simulink model "Correccion_Sist_Fisico"  (R2021a)
settings: Solver=VariableStepAuto  StartTime=0.0  StopTime=inf  RelTol=1e-3
values from neighbouring files (symbols this model uses):
  b_cx = 1*10^6    (= 1000000)    [parametros.m]
  b_cy = 1*10^7    (= 10000000)    [parametros.m]
  b_eq = (b_td+b_tm*(r_t^2))/r_td    (= 10803.6)    [parametros.m]
  b_eqh = 2*(b_hd+b_hm*(r_h^2))/r_hd    (= 23253.3333333)    [parametros.m]
  b_ha = b_eqh/r_h - n_h*w_posh*(J_eqh + 0.5*m_l_*r_hd)/r_h    [parametros.m]
  b_hb = 1*10^8    (= 100000000)    [parametros.m]
  b_hEb = 2.2*10^9    (= 2200000000)    [parametros.m]
  b_t = 90    [parametros.m]
  b_ta = n_t*w_post*(r_td*J_eqt/r_t) - r_td*b_eqt/r_t    [parametros.m]
  b_tb = 5*10^6    (= 5000000)    [parametros.m]
  b_tw = 3*10^3    (= 3000)    [parametros.m]
  b_wu = 150    [parametros.m]
  g = 9.80665    [parametros.m]
  H_c = 2.5    [parametros.m]
  J_eq = (J_td+J_tm_tb*(r_t^2))/r_td    (= 15000)    [parametros.m]
  J_eqh = 2*(J_hd_hEb+J_hm_hb*(r_h^2))/r_hd    (= 48853.3333333)    [parametros.m]
  K_cy = 1.8*10^9    (= 1800000000)    [parametros.m]
  K_hsa = -n_h*(w_posh^2)*(J_eqh + 0.5*m_l_*r_hd)/r_t    [parametros.m]
  K_hsia = -(w_posh^3)*(J_eqh + 0.5*m_l_*r_hd)/r_t    [parametros.m]
  K_tsa = n_t*(w_post^2)*J_eqt*r_td/r_t    [parametros.m]
  K_tsia = (w_post^3)*J_eqt*r_td/r_t    [parametros.m]
  K_tw = 4.8*10^5    (= 480000)    [parametros.m]
  k_wu = 2.36*10^8    (= 236000000)    [parametros.m]
  lh_inicial = 45-yl_inicial    (= 40)    [parametros.m]
  M_c_MAX = 50000 + M_s    (= 65000)    [parametros.m]
  M_real = 10000    [parametros.m]
  M_s = 15000    [parametros.m]
  M_t = 30000    [parametros.m]
  r_h = 22    [parametros.m]
  r_hd = 0.75    [parametros.m]
  r_t = 30    [parametros.m]
  r_td = 0.5    [parametros.m]
  T_hb_MAX = 5*10^4    (= 50000)    [parametros.m]
  T_hEb_MAX = 1.1*10^6    (= 1100000)    [parametros.m]
  T_hm_MAX = 2*10^4    (= 20000)    [parametros.m]
  T_s2 = 5e-3    (= 0.005)    [parametros.m]
  T_tb_MAX = 5*10^3    (= 5000)    [parametros.m]
  T_tm_MAX = 3*10^3    (= 3000)    [parametros.m]
  tau_hm = 1.0e-2    (= 0.01)    [parametros.m]
  tau_tm = 1.0e-2    (= 0.01)    [parametros.m]
  TensionMinima = (M_s*g/2)*0.5    (= 36774.9375)    [parametros.m]
  v_h_MAX_c = +1.5    (= 1.5)    [parametros.m]
  v_t_MAX = +4    (= 4)    [parametros.m]
  v_t_MIN = -4    [parametros.m]
  w_hm_min = pi/4    (= 0.785398163397)    [parametros.m]
  w_tm_min = pi/4    (= 0.785398163397)    [parametros.m]
  xt_inicial = -10    [parametros.m]
  Y_t0 = 45    [parametros.m]
  yl_inicial = 5    [parametros.m]
undefined symbols (not defined in the file or in its folder): DiscIntNeverNeededParam
libraries: simulink x10, dspstat3 x1, vrlib x1
(part 1 of 3)
settings Model: Creator=aguss  LastModifiedBy=aguss
settings SolverCC: ZeroCrossAlgorithm=Adaptive
settings DebuggingCC: IgnoredZcDiagnostic=none

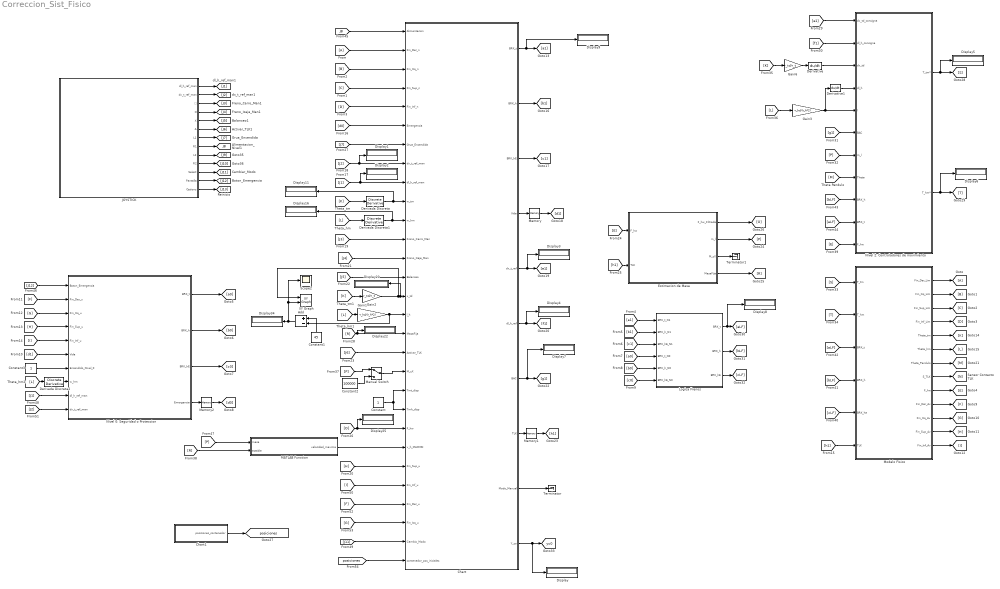
== system Correccion_Sist_Fisico ==
  Add : Sum  Inputs=+-
  Chart : Stateflow chart  TreatAsAtomicUnit=on
      settings: PortSchema="{\"entries\":[{\"content\":{\"sides\":[{\"content\":{\"connectorIds\":[\"In1\",\"In2\",\"In3\",\"In4\",\"In5\",\"In6\",\"In7\",\"In8\",\"In9\",\"In10\",\"In11\",\"In12\",\"In13\",\"In14\",\"In15\",\"In16\",\"In17\",\"In18\",\"In19\",\"In20\",\"In21\",\"In22\",\"In23\",\"In24\",\"In25\",\"In28\",\"In27\",\"In26\",\"In29\"]},\"type\":\"ConnectorPlacement.EquallySpacedRectSide\",\"uuid\":\"54a235bb-383c-4b33-a4d9-6e61ae54fc2f\"},{\"content\":{\"connectorIds\":[\"Out1\",\"Out2\",\"Out3\",\"Out4\",\"Out5\",\"Out6\",\"Out7\",\"Out8\",\"Out9\",\"Out10\"],\"side\":\"RIGHT\"},\"type\":\"ConnectorPlacement.EquallySpacedRectSide\",\"uuid\":\"22d5bc5e-44c7-4d0f-b301-3d6b5a5c05fa\"},{\"content\":{\"connectorIds\":[],\"side\":\"TOP\"},\"type\":\"ConnectorPlacement.EquallySpacedRectSide\",\"uuid\":\"f8e7191e-c2be-47a5-9ee2-638adab41de6\"},{\"content\":{\"connectorIds\":[],\"side\":\"BOTTOM\"},\"type\":\"ConnectorPlacement.EquallySpacedRectSide\",\"uuid\":\"c3fe6b96-a7cd-4655-bccb-6e03a1555df7\"}]},\"type\":\"ConnectorPlacement.EquallySpacedConnector\",\"uuid\":\"917daf47-55d7-4e55-b1eb-670cdd820ed3\"}],\"packageUris\":[\"http://schema.mathworks.com/mf0/Connector/R2020b\"],\"version\":\"1.0\"}"
  Chart1 : Stateflow chart  TreatAsAtomicUnit=on
  Constant : Constant
  Constant1 : Constant  Value=45
  Constant2 : Constant  Value=100000
  Constant3 : Constant
  Derivada Discreta : simulink/Discrete/Discrete Derivative  gainval=1.0  ICPrevScaledInput=0.0  OutMin=[]  OutMax=[]  OutDataType=fixdt(1, 16)  OutScaling=2^-10  DoSatur=off
  Derivada Discreta1 : simulink/Discrete/Discrete Derivative  gainval=1.0  ICPrevScaledInput=0.0  OutMin=[]  OutMax=[]  OutDataType=fixdt(1, 16)  OutScaling=2^-10  DoSatur=off
  Derivada Discreta2 : simulink/Discrete/Discrete Derivative  gainval=1.0  ICPrevScaledInput=0.0  OutMin=[]  OutMax=[]  OutDataType=fixdt(1, 16)  OutScaling=2^-10  DoSatur=off
  Derivative : Derivative
  Derivative1 : Derivative
  Display{,1..9,11,16,20,22,25,34} (16 alike) : Display
  Estimacion de Masa : Subsystem
  Gain1 : Gain  Gain=-r_hd/(r_h*2)
  Gain2 : Gain  Gain=r_td/r_t
  Gain3 : Gain  Gain=-r_hd/(r_h*2)
  Gain6 : Gain  Gain=r_td/r_t
  JOYSTICK : Subsystem
  Logica Frenos : Subsystem
  MATLAB Function : MATLAB Function  TreatAsAtomicUnit=on
  Manual Switch : ManualSwitch
  Memory : Memory
  Memory1 : Memory
  Memory2 : Memory
  Modelo Físico : Subsystem
  Nivel 0: Seguridad o Proteccion : Stateflow chart  TreatAsAtomicUnit=on
  Nivel 2: Controladores de movimiento : Subsystem
  Scope2 : Scope
  Terminator : Terminator
  Terminator1 : Terminator
  XY Graph : simulink/Sinks/XY Graph  xmin=-32  xmax=52  ymin=-22  ymax=42  st=-1
  tag scope: J8=global, posiciones=global, yc0=global
  wires:
  Modelo Físico/5(Theta_tm) -> [K]
  Modelo Físico/6(Theta_hm) -> [L]
  Modelo Físico/10(Fin_Der_Av) -> [F]
  Modelo Físico/7(Theta_Pendulo) -> [M]
  Modelo Físico/2(Fin_Izq_Lim) -> [B]
  Modelo Físico/8(S_TLK) -> [N]
  Modelo Físico/3(Fin_Sup_Lim) -> [C]
  Modelo Físico/1(Fin_Der_Lim) -> [A]
  Modelo Físico/9(F_hw) -> [E]
  Modelo Físico/4(Fin_Inf_Lim) -> [D]
  Modelo Físico/11(Fin_Izq_Av) -> [G]
  Modelo Físico/12(Fin_Sup_Av) -> [H]
  Modelo Físico/13(Fin_Inf_Av) -> [I]
  [B] -> Chart/3(Fin_Izq_n)
  [A] -> Chart/2(Fin_Der_n)
  Constant/1 -> Chart/20(Tmt_disp), Chart/21(Tmh_disp)
  [J8] -> Chart/1(Alimentacion)
  [C] -> Chart/4(Fin_Sup_n)
  [D] -> Chart/5(Fin_Inf_n)
  [J7] -> Chart/7(Grua_Encendida)
  Derivada Discreta1/1 -> Display16/1, Chart/11(w_hm)
  Derivada Discreta/1 -> Chart/10(w_tm), Display11/1
  Gain2/1 -> Display20/1, Chart/15(x_td), XY Graph/1
  MATLAB Function/1(velocidad_maxima) -> Chart/23(v_h_MAXMIN)
  JOYSTICK/13(Options) -> [J13]
  JOYSTICK/9(L2) -> [J9]
  JOYSTICK/12(Pantalla) -> [J12]
  JOYSTICK/4(O) -> [J4]
  JOYSTICK/1(dl_h_ref_man) -> [J1]
  JOYSTICK/6(Δ) -> [J6]
  JOYSTICK/5(X) -> [J5]
  JOYSTICK/10(R2) -> [J10]
  JOYSTICK/2(dx_t_ref_man) -> [J2]
  JOYSTICK/11(Select) -> [J11]
  JOYSTICK/8(R1) -> [J8]
  JOYSTICK/3(☐) -> [J3]
  JOYSTICK/7(L1) -> [J7]
  Chart/9(Modo_Manual) -> Terminator/1
  Nivel 0: Seguridad o Proteccion/1(BRK_t) -> [a0]
  Nivel 0: Seguridad o Proteccion/2(BRK_h) -> [b0]
  Nivel 0: Seguridad o Proteccion/3(BRK_hE) -> [c0]
  Nivel 0: Seguridad o Proteccion/4(Emergencia) -> Memory2/1
  [a1] -> Logica Frenos/1(BRK_t_N1)
  [b1] -> Logica Frenos/2(BRK_h_N1)
  [c1] -> Logica Frenos/3(BRK_hE_N1)
  [a0] -> Logica Frenos/4(BRK_t_N0)
  [b0] -> Logica Frenos/5(BRK_h_N0)
  [c0] -> Logica Frenos/6(BRK_hE_N0)
  Chart/4(Vida) -> Memory/1
  [d1] -> Nivel 0: Seguridad o Proteccion/6(Vida)
  [F] -> Nivel 0: Seguridad o Proteccion/2(Fin_Der_u)
  [G] -> Nivel 0: Seguridad o Proteccion/3(Fin_Izq_u)
  [I] -> Nivel 0: Seguridad o Proteccion/5(Fin_Inf_u)
  Constant3/1 -> Nivel 0: Seguridad o Proteccion/7(Encendido_Nivel_0)
  Chart/8(TLK) -> Memory1/1
  [h1] -> Modelo Físico/6(TLK)
  [E] -> Estimacion de Masa/1(F_hw)
  [h1] -> Estimacion de Masa/2(TLK)
  Estimacion de Masa/2(m_l) -> [P]
  [f1] -> Nivel 2: Controladores de movimiento/2(dl_h_consigna)
  [e1] -> Nivel 2: Controladores de movimiento/1(dx_td_consigna)
  [g1] -> Nivel 2: Controladores de movimiento/6(BAC)
  [P] -> Nivel 2: Controladores de movimiento/7(m_l)
  Nivel 2: Controladores de movimiento/2(T_hm*) -> Display6/1, [T]
  Nivel 2: Controladores de movimiento/1(T_tm*) -> Display5/1, [S]
  [S] -> Modelo Físico/1(T_tm)
  [T] -> Modelo Físico/2(T_hm)
  [K] -> Gain6/1
  Gain6/1 -> Derivative/1
  [L] -> Gain3/1
  Gain3/1 -> Derivative1/1, Nivel 2: Controladores de movimiento/5(l)
  Derivative1/1 -> Nivel 2: Controladores de movimiento/4(dl_h)
  [M] -> Nivel 2: Controladores de movimiento/8(Theta)
  Memory/1 -> [d1]
  Memory1/1 -> [h1]
  Memory2/1 -> [d0]
  Estimacion de Masa/4(MasaFija) -> [R]
  Chart/6(dl_h_ref) -> Display4/1, [f1]
  Chart/5(dx_t_ref) -> Display3/1, [e1]
  [P] -> MATLAB Function/1(masa)
  [K] -> Derivada Discreta/1
  [d0] -> Chart/6(Emergencia)
  [J1] -> Display2/1, Chart/9(dl_h_ref_man)
  [J2] -> Display1/1, Chart/8(dx_t_ref_man)
  [J5] -> Chart/14(Balanceo)
  [L] -> Derivada Discreta1/1
  [J4] -> Chart/13(Freno_Izaje_Man)
  [J3] -> Chart/12(Freno_Carro_Man)
  [J6] -> Chart/18(Activar_TLK)
  [K] -> Gain2/1
  [R] -> Chart/17(MasaFija), Display22/1
  [L] -> Gain1/1
  [O] -> Chart/22(F_hw), Display25/1
  Chart/7(BAC) -> Display7/1, [g1]
  Chart/3(BRK_hE) -> [c1]
  Chart/2(BRK_h) -> [b1]
  [P] -> Manual Switch/1
  [R] -> MATLAB Function/2(estable)
  [E] -> Nivel 2: Controladores de movimiento/11(F_hw)
  Logica Frenos/1(BRK_t) -> Display8/1, [aLF]
  Logica Frenos/2(BRK_h) -> [bLF]
  Logica Frenos/3(BRK_hE) -> [cLF]
  [aLF] -> Modelo Físico/3(BRK_t)
  [bLF] -> Modelo Físico/4(BRK_h)
  [cLF] -> Modelo Físico/5(BRK_he)
  [aLF] -> Nivel 2: Controladores de movimiento/10(BRK_t)
  [bLF] -> Nivel 2: Controladores de movimiento/9(BRK_h)
  [J12] -> Nivel 0: Seguridad o Proteccion/1(Boton_Emergencia)
  [L] -> Derivada Discreta2/1
  Derivada Discreta2/1 -> Nivel 0: Seguridad o Proteccion/8(w_hm)
  Gain1/1 -> Chart/16(l_h), Add/2
  Add/1 -> XY Graph/2, Scope2/1, Display34/1
  Constant1/1 -> Add/1
  [H] -> Nivel 0: Seguridad o Proteccion/4(Fin_Sup_u)
  [H] -> Chart/24(Fin_Sup_u)
  [J1] -> Nivel 0: Seguridad o Proteccion/9(dl_h_ref_man)
  [J11] -> Chart/26(Cambio_Modo)
  [I] -> Chart/25(Fin_Inf_u)
  [J2] -> Nivel 0: Seguridad o Proteccion/10(dx_t_ref_man)
  [F] -> Chart/28(Fin_Der_u)
  [G] -> Chart/27(Fin_Izq_u)
  Derivative/1 -> Nivel 2: Controladores de movimiento/3(dx_td)
  Manual Switch/1 -> Chart/19(M_cX)
  Constant2/1 -> Manual Switch/2
  Estimacion de Masa/1(F_hw_Filtrada) -> [O]
  Estimacion de Masa/3(M_cX) -> Terminator1/1
  Chart1/1(posiciones_contenedor) -> [posiciones]
  [posiciones] -> Chart/29(contenedor_pos_iniciales)
  Chart/10(Y_co) -> Display/1, [yc0]
  Chart/1(BRK_t) -> Display9/1, [a1]

== system Correccion_Sist_Fisico/Estimacion de Masa ==
  F_hw : Inport
  TLK : Inport  Port=2
  Discrete Derivative1 : simulink/Discrete/Discrete Derivative  gainval=1.0  ICPrevScaledInput=0.0  OutMin=[]  OutMax=[]  OutDataType=fixdt(1, 16)  OutScaling=2^-10  DoSatur=off
  Leaky integrator : Subsystem
  MATLAB Function1 : MATLAB Function  TreatAsAtomicUnit=on
  Moving Average2 : dspstat3/Moving Average  Method=Sliding window  ForgettingFactorPort=off  SpecifyWindowLength=on  WindowLength=4  ForgettingFactor=0.9  SimulateUsing=Code generation
  Zero-Order Hold : ZeroOrderHold  SampleTime=-1
  F_hw_Filtrada : Outport
  m_l : Outport  Port=2
  M_cX : Outport  Port=3
  MasaFija : Outport  Port=4
  wires:
  Moving Average2/1 -> Discrete Derivative1/1, Zero-Order Hold/1
  Discrete Derivative1/1 -> MATLAB Function1/2(dF_hw)
  TLK/1 -> MATLAB Function1/3(TLK)
  F_hw/1 -> Leaky integrator/1(Entrada)
  MATLAB Function1/1(m_l) -> m_l/1
  MATLAB Function1/2(M_cX) -> M_cX/1
  MATLAB Function1/3(MasaFija) -> MasaFija/1
  Leaky integrator/1(Salida) -> Moving Average2/1
  Zero-Order Hold/1 -> F_hw_Filtrada/1, MATLAB Function1/1(tension)

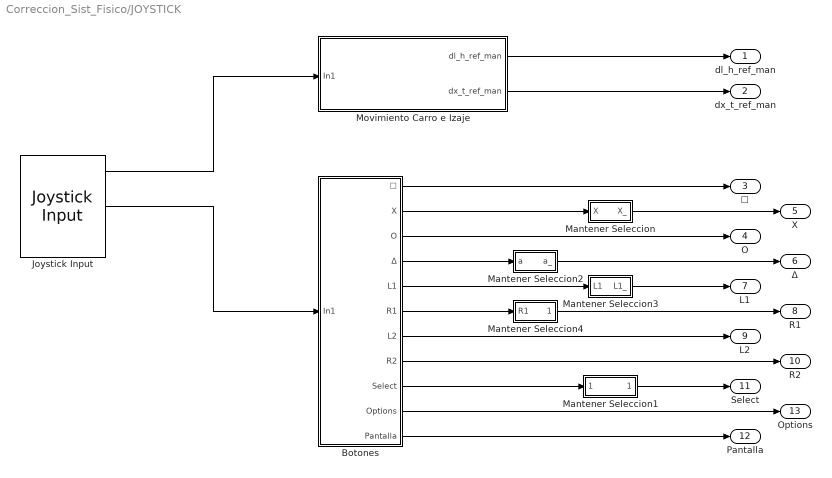
== system Correccion_Sist_Fisico/JOYSTICK ==
  Botones : Subsystem
  Joystick Input : vrlib/Joystick Input  joyid=1  adjustports=on  forcefeed=off
  Mantener Seleccion : Stateflow chart  TreatAsAtomicUnit=on
  Mantener Seleccion1 : Stateflow chart  TreatAsAtomicUnit=on
  Mantener Seleccion2 : Stateflow chart  TreatAsAtomicUnit=on
  Mantener Seleccion3 : Stateflow chart  TreatAsAtomicUnit=on
  Mantener Seleccion4 : Stateflow chart  TreatAsAtomicUnit=on
  Movimiento Carro e Izaje : Subsystem
  dl_h_ref_man : Outport
  dx_t_ref_man : Outport  Port=2
  ☐ : Outport  Port=3
  O : Outport  Port=4
  X : Outport  Port=5
  Δ : Outport  Port=6
  L1 : Outport  Port=7
  R1 : Outport  Port=8
  L2 : Outport  Port=9
  R2 : Outport  Port=10
  Select : Outport  Port=11
  Pantalla : Outport  Port=12
  Options : Outport  Port=13
  wires:
  Joystick Input/1 -> Movimiento Carro e Izaje/1(In1)
  Movimiento Carro e Izaje/1(dl_h_ref_man) -> dl_h_ref_man/1
  Movimiento Carro e Izaje/2(dx_t_ref_man) -> dx_t_ref_man/1
  Joystick Input/2 -> Botones/1(In1)
  Botones/1(☐) -> ☐/1
  Botones/2(X) -> Mantener Seleccion/1(X)
  Botones/3(O) -> O/1
  Botones/4(Δ) -> Mantener Seleccion2/1(a)
  Botones/5(L1) -> Mantener Seleccion3/1(L1)
  Botones/6(R1) -> Mantener Seleccion4/1(R1)
  Botones/7(L2) -> L2/1
  Botones/8(R2) -> R2/1
  Botones/9(Select) -> Mantener Seleccion1/1(Select)
  Botones/10(Options) -> Options/1
  Botones/11(Pantalla) -> Pantalla/1
  Mantener Seleccion/1(X_) -> X/1
  Mantener Seleccion2/1(a_) -> Δ/1
  Mantener Seleccion3/1(L1_) -> L1/1
  Mantener Seleccion4/1(R1_) -> R1/1
  Mantener Seleccion1/1(Select_) -> Select/1

== system Correccion_Sist_Fisico/Logica Frenos ==
  BRK_t_N1 : Inport
  BRK_h_N1 : Inport  Port=2
  BRK_hE_N1 : Inport  Port=3
  BRK_t_N0 : Inport  Port=4
  BRK_h_N0 : Inport  Port=5
  BRK_hE_N0 : Inport  Port=6
  AND : Logic  IconShape=distinctive  AllPortsSameDT=off  OutDataTypeStr=boolean
  AND1 : Logic  IconShape=distinctive  AllPortsSameDT=off  OutDataTypeStr=boolean
  AND2 : Logic  IconShape=distinctive  AllPortsSameDT=off  OutDataTypeStr=boolean
  BRK_t : Outport
  BRK_h : Outport  Port=2
  BRK_hE : Outport  Port=3
  wires:
  AND/1 -> BRK_h/1
  BRK_h_N1/1 -> AND/1
  BRK_h_N0/1 -> AND/2
  AND1/1 -> BRK_t/1
  BRK_t_N1/1 -> AND1/1
  BRK_t_N0/1 -> AND1/2
  AND2/1 -> BRK_hE/1
  BRK_hE_N1/1 -> AND2/1
  BRK_hE_N0/1 -> AND2/2

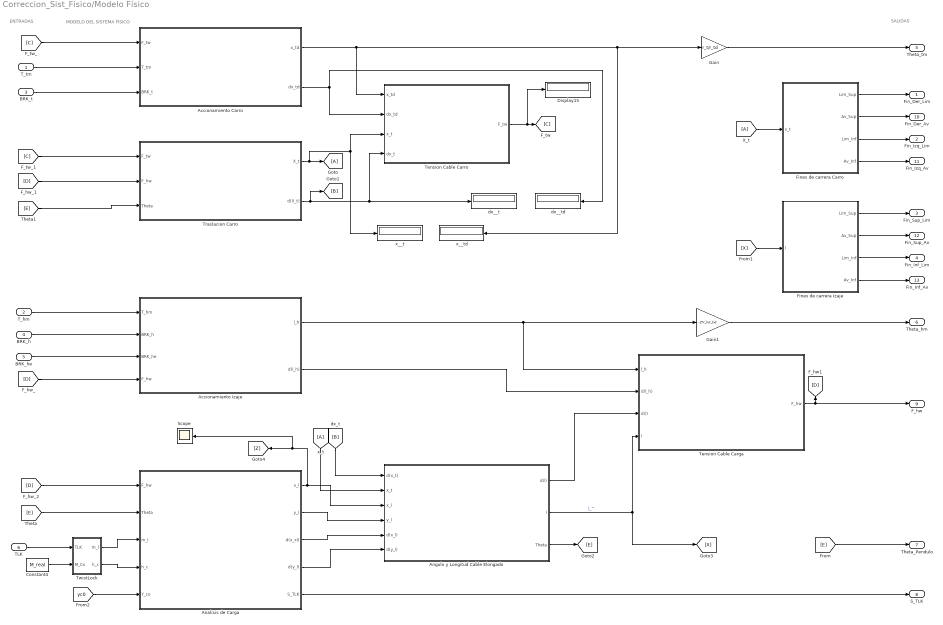
== system Correccion_Sist_Fisico/Modelo Físico ==
  note: SALIDAS
  note: MODELO DEL SISTEMA FÍSICO
  note: ENTRADAS
  T_tm : Inport
  T_hm : Inport  Port=2
  BRK_t : Inport  Port=3
  BRK_h : Inport  Port=4
  BRK_he : Inport  Port=5
  TLK : Inport  Port=6
  Accionamiento Carro : Subsystem
  Accionamiento Izaje : Subsystem
  Analisis de Carga : Subsystem
  Angulo y Longitud Cable Elongado : Subsystem
  Constant4 : Constant  Value=M_real
  Display15 : Display
  Fines de carrera Carro : Subsystem
  Fines de carrera Izaje : Subsystem
  Gain : Gain  Gain=r_t/r_td
  Gain1 : Gain  Gain=-2*r_h/r_hd
  Scope : Scope
  Tension Cable Carga : Subsystem
  Tension Cable Carro : Subsystem
  Traslacion Carro : Subsystem
  TwistLock : Subsystem
  dx__t : Display
  dx__td : Display
  x__t : Display
  x__td : Display
  Fin_Der_Lim : Outport
  Fin_Izq_Lim : Outport  Port=2
  Fin_Sup_Lim : Outport  Port=3
  Fin_Inf_Lim : Outport  Port=4
  Theta_tm : Outport  Port=5
  Theta_hm : Outport  Port=6
  Theta_Pendulo : Outport  Port=7
  S_TLK : Outport  Port=8
  F_hw : Outport  Port=9
  Fin_Der_Av : Outport  Port=10
  Fin_Izq_Av : Outport  Port=11
  Fin_Sup_Av : Outport  Port=12
  Fin_Inf_Av : Outport  Port=13
  wires:
  Analisis de Carga/5(S_TLK) -> S_TLK/1
  Fines de carrera Carro/3(Lim_Inf) -> Fin_Izq_Lim/1
  Traslacion Carro/1(X_t) -> Tension Cable Carro/3(x_t), x__t/1, [A]
  Fines de carrera Izaje/2(Av_Sup) -> Fin_Sup_Av/1
  [D] -> Accionamiento Izaje/4(F_hw)
  Angulo y Longitud Cable Elongado/3(Theta) -> [E]
  T_tm/1 -> Accionamiento Carro/2(T_tm)
  Tension Cable Carga/1(F_hw) -> F_hw/1, [D]
  TwistLock/1(m_l) -> Analisis de Carga/3(m_l)
  [E] -> Analisis de Carga/2(Theta)
  Accionamiento Izaje/1(l_h) -> Gain1/1, Tension Cable Carga/1(l_h)
  BRK_t/1 -> Accionamiento Carro/3(BRK_t)
  Fines de carrera Carro/1(Lim_Sup) -> Fin_Der_Lim/1
  Accionamiento Carro/1(x_td) -> x__td/1, Gain/1, Tension Cable Carro/1(x_td)
  Fines de carrera Izaje/3(Lim_Inf) -> Fin_Inf_Lim/1
  Analisis de Carga/2(y_l) -> Angulo y Longitud Cable Elongado/4(y_l)
  TwistLock/2(h_c) -> Analisis de Carga/4(h_c)
  BRK_h/1 -> Accionamiento Izaje/2(BRK_h)
  Fines de carrera Carro/2(Av_Sup) -> Fin_Der_Av/1
  [D] -> Analisis de Carga/1(F_hw)
  Accionamiento Carro/2(dx_td) -> Tension Cable Carro/2(dx_td), dx__td/1
  Tension Cable Carro/1(F_tw) -> Display15/1, [C]
  T_hm/1 -> Accionamiento Izaje/1(T_hm)
  [C] -> Accionamiento Carro/1(F_tw)
  [E] -> Theta_Pendulo/1
  Traslacion Carro/2(d(X_t)) -> Tension Cable Carro/4(dx_t), dx__t/1, [B]
  [D] -> Traslacion Carro/2(F_hw)
  Fines de carrera Izaje/4(Av_Inf) -> Fin_Inf_Av/1
  Angulo y Longitud Cable Elongado/1(d(l)) -> Tension Cable Carga/3(d(l))
  TLK/1 -> TwistLock/1(TLK)
  [E] -> Traslacion Carro/3(Theta)
  Accionamiento Izaje/2(d(l_h)) -> Tension Cable Carga/2(d(l_h))
  Fines de carrera Izaje/1(Lim_Sup) -> Fin_Sup_Lim/1
  Gain1/1 -> Theta_hm/1
  Fines de carrera Carro/4(Av_Inf) -> Fin_Izq_Av/1
  [B] -> Angulo y Longitud Cable Elongado/1(d(x_t))
  Analisis de Carga/3(d(x_xl)) -> Angulo y Longitud Cable Elongado/5(d(x_l))
  Analisis de Carga/4(d(y_l)) -> Angulo y Longitud Cable Elongado/6(d(y_l))
  Gain/1 -> Theta_tm/1
  [C] -> Traslacion Carro/1(F_tw)
  [A] -> Angulo y Longitud Cable Elongado/2(x_t)
  [A] -> Fines de carrera Carro/1(x_t)
  BRK_he/1 -> Accionamiento Izaje/3(BRK_he)
  [X] -> Fines de carrera Izaje/1(l)
  Analisis de Carga/1(x_l) -> Angulo y Longitud Cable Elongado/3(x_l), Scope/1, [Z]
  Angulo y Longitud Cable Elongado/2(l) -> Tension Cable Carga/4(l), [X]  "l_^"
  Constant4/1 -> TwistLock/2(M_Cx)
  [yc0] -> Analisis de Carga/5(Y_co)

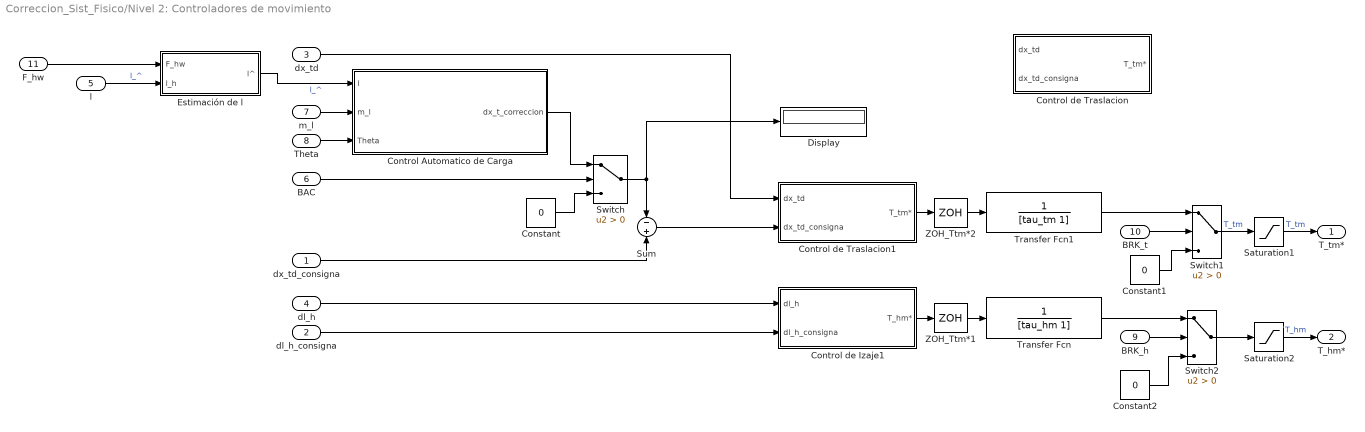
== system Correccion_Sist_Fisico/Nivel 2: Controladores de movimiento ==
  dx_td_consigna : Inport
  dl_h_consigna : Inport  Port=2
  dx_td : Inport  Port=3
  dl_h : Inport  Port=4
  l : Inport  Port=5
  BAC : Inport  Port=6
  m_l : Inport  Port=7
  Theta : Inport  Port=8
  BRK_h : Inport  Port=9
  BRK_t : Inport  Port=10
  F_hw : Inport  Port=11
  Constant : Constant  Value=0
  Constant1 : Constant  Value=0
  Constant2 : Constant  Value=0
  Control Automatico de Carga : Subsystem
  Control de Izaje1 : Subsystem
  Control de Traslacion : Subsystem
  Control de Traslacion1 : Subsystem
  Display : Display
  Estimación de l : Subsystem
  Saturation1 : Saturate  UpperLimit=T_tm_MAX  LowerLimit=-T_tm_MAX
  Saturation2 : Saturate  UpperLimit=T_hm_MAX  LowerLimit=-T_hm_MAX
  Sum : Sum  Inputs=-+
  Switch : Switch  Criteria=u2 > Threshold
  Switch1 : Switch  Criteria=u2 > Threshold
  Switch2 : Switch  Criteria=u2 > Threshold
  Transfer Fcn : TransferFcn  Denominator=[tau_hm 1]
  Transfer Fcn1 : TransferFcn  Denominator=[tau_tm 1]
  ZOH_Ttm*1 : ZeroOrderHold  SampleTime=T_s2
  ZOH_Ttm*2 : ZeroOrderHold  SampleTime=T_s2
  T_tm* : Outport
  T_hm* : Outport  Port=2
  wires:
  Control de Izaje1/1(T_hm*) -> ZOH_Ttm*1/1
  dx_td_consigna/1 -> Sum/2
  dx_td/1 -> Control de Traslacion1/1(dx_td)
  dl_h/1 -> Control de Izaje1/1(dl_h)
  dl_h_consigna/1 -> Control de Izaje1/2(dl_h_consigna)
  Sum/1 -> Control de Traslacion1/2(dx_td_consigna)
  Control Automatico de Carga/1(dx_t_correccion) -> Switch/1
  Constant/1 -> Switch/3
  Switch/1 -> Sum/1, Display/1
  BAC/1 -> Switch/2
  Theta/1 -> Control Automatico de Carga/3(Theta)
  m_l/1 -> Control Automatico de Carga/2(m_l)
  Transfer Fcn1/1 -> Switch1/1
  Switch2/1 -> Saturation2/1
  Switch1/1 -> Saturation1/1  "T_tm"
  Transfer Fcn/1 -> Switch2/1
  BRK_h/1 -> Switch2/2
  BRK_t/1 -> Switch1/2
  Saturation2/1 -> T_hm*/1  "T_hm"
  F_hw/1 -> Estimación de l/1(F_hw)
  l/1 -> Estimación de l/2(l_h)  "l_^"
  Estimación de l/1(l^) -> Control Automatico de Carga/1(l)  "l_^"
  Constant1/1 -> Switch1/3
  Constant2/1 -> Switch2/3
  Control de Traslacion1/1(T_tm*) -> ZOH_Ttm*2/1
  ZOH_Ttm*1/1 -> Transfer Fcn/1
  ZOH_Ttm*2/1 -> Transfer Fcn1/1
  Saturation1/1 -> T_tm*/1  "T_tm"

== system Correccion_Sist_Fisico/Estimacion de Masa/Leaky integrator ==
  Entrada : Inport
  Constant17 : Constant
  Delay1 : Delay  DelayLength=1  InitialCondition=0
  Divide1 : Product  Inputs=*/
  M : Constant  Value=100
  Product2 : Product
  Product3 : Product
  Sum1 : Sum  Inputs=|+-
  Sum2 : Sum  Inputs=|-+
  Sum5 : Sum  Inputs=|++
  Salida : Outport
  wires:
  Sum5/1 -> Salida/1, Delay1/1
  M/1 -> Sum2/2, Divide1/2
  Constant17/1 -> Sum2/1, Sum1/1
  Sum1/1 -> Product2/2
  Product2/1 -> Sum5/1
  Delay1/1 -> Product3/1
  Divide1/1 -> Product3/2, Sum1/2
  Product3/1 -> Sum5/2
  Sum2/1 -> Divide1/1
  Entrada/1 -> Product2/1

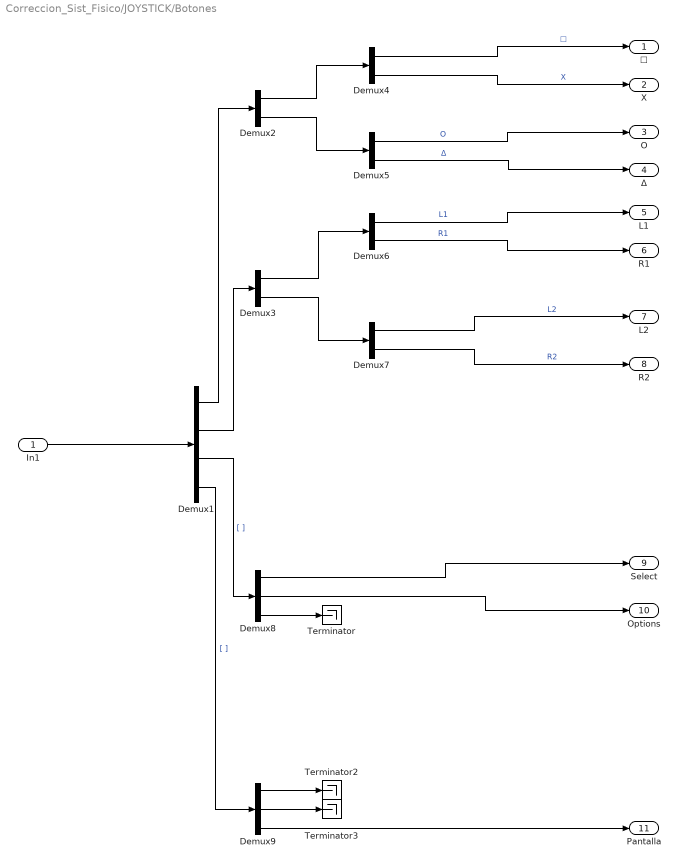
== system Correccion_Sist_Fisico/JOYSTICK/Botones ==
  In1 : Inport
  Demux1 : Demux
  Demux{2..7} (6 alike) : Demux  Outputs=2
  Demux8 : Demux  Outputs=3
  Demux9 : Demux  Outputs=3
  Terminator : Terminator
  Terminator2 : Terminator
  Terminator3 : Terminator
  ☐ : Outport
  X : Outport  Port=2
  O : Outport  Port=3
  Δ : Outport  Port=4
  L1 : Outport  Port=5
  R1 : Outport  Port=6
  L2 : Outport  Port=7
  R2 : Outport  Port=8
  Select : Outport  Port=9
  Options : Outport  Port=10
  Pantalla : Outport  Port=11
  wires:
  Demux6/1 -> L1/1  "L1"
  Demux7/2 -> R2/1  "R2"
  Demux1/2 -> Demux3/1
  Demux1/1 -> Demux2/1
  Demux2/1 -> Demux4/1
  Demux3/2 -> Demux7/1
  Demux2/2 -> Demux5/1
  Demux3/1 -> Demux6/1
  Demux7/1 -> L2/1  "L2"
  Demux4/1 -> ☐/1  "☐"
  Demux5/2 -> Δ/1  "Δ"
  Demux5/1 -> O/1  "O"
  Demux6/2 -> R1/1  "R1"
  Demux4/2 -> X/1  "X"
  Demux1/3 -> Demux8/1  "[ ]"
  In1/1 -> Demux1/1
  Demux8/1 -> Select/1
  Demux8/2 -> Options/1
  Demux8/3 -> Terminator/1
  Demux9/3 -> Pantalla/1
  Demux1/4 -> Demux9/1  "[ ]"
  Demux9/1 -> Terminator2/1
  Demux9/2 -> Terminator3/1

== system Correccion_Sist_Fisico/JOYSTICK/Movimiento Carro e Izaje ==
  In1 : Inport
  Demux : Demux  Outputs=5
  Demux8 : Demux  Outputs=2
  Sensibilidad1 : Subsystem
  Terminator{,2..4} (4 alike) : Terminator
  dl_h_ref_man : Outport
  dx_t_ref_man : Outport  Port=2
  wires:
  Demux8/2 -> Sensibilidad1/1(Analogo_IZQ_Vertical)  "AI_V"
  Demux/3 -> Terminator2/1  "L2"
  Demux/4 -> Terminator3/1  "R2"
  Sensibilidad1/1(dl_h_ref_manual) -> dl_h_ref_man/1
  Sensibilidad1/2(dx_t_ref_man) -> dx_t_ref_man/1
  Demux/5 -> Terminator4/1  "AD_V"
  Demux8/1 -> Terminator/1  "AI_H"
  Demux/1 -> Demux8/1
  In1/1 -> Demux/1
  Demux/2 -> Sensibilidad1/2(Analogo_DER_Horizontal)  "AI_V"

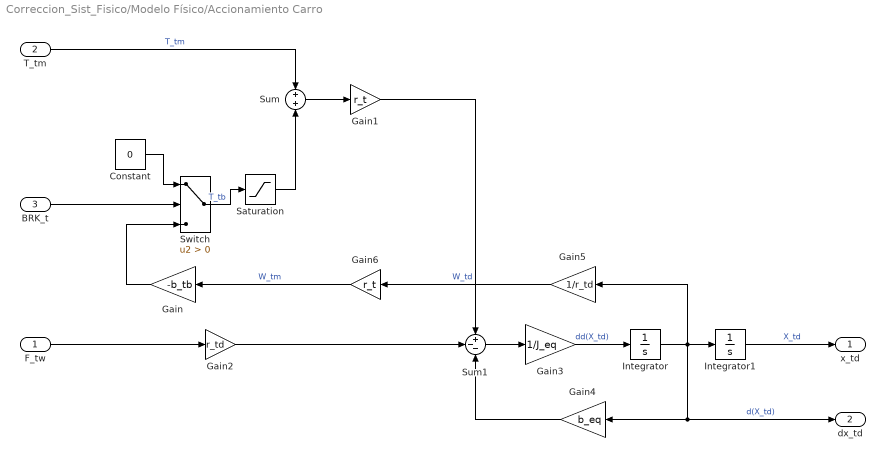
== system Correccion_Sist_Fisico/Modelo Físico/Accionamiento Carro ==
  F_tw : Inport
  T_tm : Inport  Port=2
  BRK_t : Inport  Port=3
  Constant : Constant  Value=0
  Gain : Gain  Gain=-b_tb
  Gain1 : Gain  Gain=r_t
  Gain2 : Gain  Gain=r_td
  Gain3 : Gain  Gain=1/J_eq
  Gain4 : Gain  Gain=b_eq
  Gain5 : Gain  Gain=1/r_td
  Gain6 : Gain  Gain=r_t
  Integrator : Integrator
  Integrator1 : Integrator  InitialCondition=xt_inicial
  Saturation : Saturate  UpperLimit=T_tb_MAX  LowerLimit=-T_tb_MAX
  Sum : Sum
  Sum1 : Sum  Inputs=+--
  Switch : Switch  Criteria=u2 > Threshold
  x_td : Outport
  dx_td : Outport  Port=2
  wires:
  BRK_t/1 -> Switch/2
  Gain/1 -> Switch/3
  Switch/1 -> Saturation/1  "T_tb"
  T_tm/1 -> Sum/1  "T_tm"
  Sum/1 -> Gain1/1
  Gain1/1 -> Sum1/1
  F_tw/1 -> Gain2/1
  Gain2/1 -> Sum1/2
  Sum1/1 -> Gain3/1
  Gain3/1 -> Integrator/1  "dd(X_td)"
  Integrator/1 -> Gain5/1, dx_td/1, Gain4/1, Integrator1/1  "d(X_td)"
  Integrator1/1 -> x_td/1  "X_td"
  Gain4/1 -> Sum1/3
  Gain5/1 -> Gain6/1  "W_td"
  Gain6/1 -> Gain/1  "W_tm"
  Saturation/1 -> Sum/2
  Constant/1 -> Switch/1

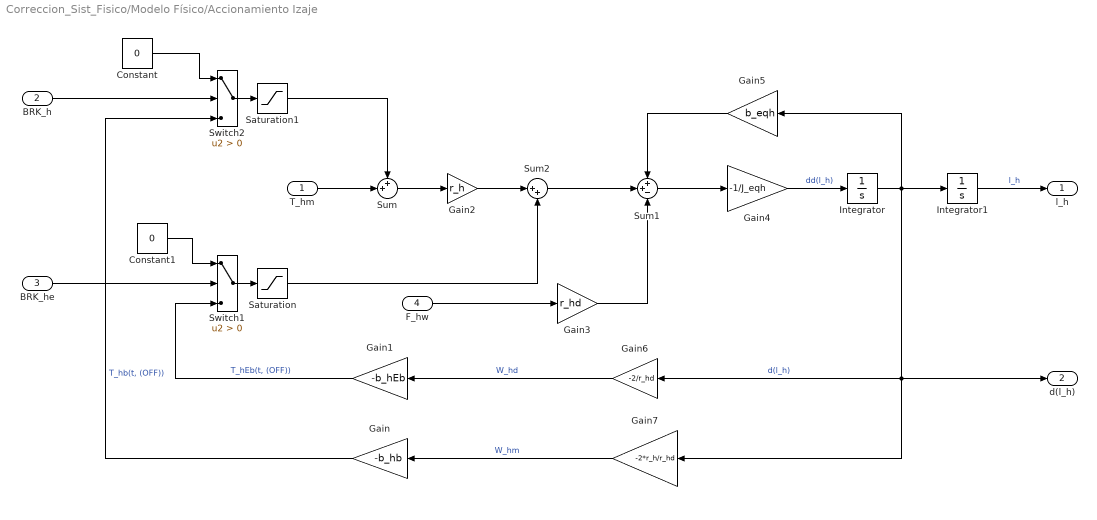
== system Correccion_Sist_Fisico/Modelo Físico/Accionamiento Izaje ==
  T_hm : Inport
  BRK_h : Inport  Port=2
  BRK_he : Inport  Port=3
  F_hw : Inport  Port=4
  Constant : Constant  Value=0
  Constant1 : Constant  Value=0
  Gain : Gain  Gain=-b_hb
  Gain1 : Gain  Gain=-b_hEb
  Gain2 : Gain  Gain=r_h
  Gain3 : Gain  Gain=r_hd
  Gain4 : Gain  Gain=-1/J_eqh
  Gain5 : Gain  Gain=b_eqh
  Gain6 : Gain  Gain=-2/r_hd
  Gain7 : Gain  Gain=-2*r_h/r_hd
  Integrator : Integrator
  Integrator1 : Integrator  InitialCondition=lh_inicial
  Saturation : Saturate  UpperLimit=T_hEb_MAX  LowerLimit=-T_hEb_MAX
  Saturation1 : Saturate  UpperLimit=T_hb_MAX  LowerLimit=-T_hb_MAX
  Sum : Sum  Inputs=++|
  Sum1 : Sum  Inputs=++-
  Sum2 : Sum  Inputs=|++
  Switch1 : Switch  Criteria=u2 > Threshold
  Switch2 : Switch  Criteria=u2 > Threshold
  l_h : Outport
  d(l_h) : Outport  Port=2
  wires:
  BRK_h/1 -> Switch2/2
  BRK_he/1 -> Switch1/2
  Gain/1 -> Switch2/3  "T_hb(t, (OFF))"
  Gain1/1 -> Switch1/3  "T_hEb(t, (OFF))"
  T_hm/1 -> Sum/2
  Switch2/1 -> Saturation1/1
  Switch1/1 -> Saturation/1
  Sum/1 -> Gain2/1
  Gain2/1 -> Sum2/1
  F_hw/1 -> Gain3/1
  Gain3/1 -> Sum1/3
  Sum1/1 -> Gain4/1
  Gain4/1 -> Integrator/1  "dd(l_h)"
  Integrator/1 -> d(l_h)/1, Gain7/1, Gain6/1, Integrator1/1, Gain5/1  "d(l_h)"
  Gain5/1 -> Sum1/1
  Gain6/1 -> Gain1/1  "W_hd"
  Gain7/1 -> Gain/1  "W_hm"
  Integrator1/1 -> l_h/1  "l_h"
  Saturation/1 -> Sum2/2
  Saturation1/1 -> Sum/1
  Sum2/1 -> Sum1/2
  Constant/1 -> Switch2/1
  Constant1/1 -> Switch1/1

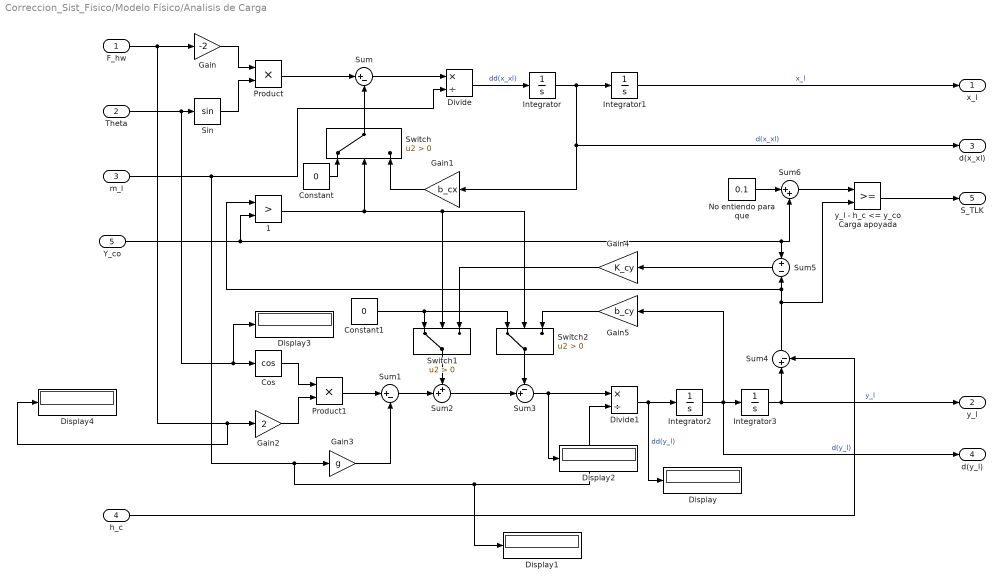
== system Correccion_Sist_Fisico/Modelo Físico/Analisis de Carga ==
  F_hw : Inport
  Theta : Inport  Port=2
  m_l : Inport  Port=3
  h_c : Inport  Port=4
  Y_co : Inport  Port=5
  1 : RelationalOperator  Operator=>  OutDataTypeStr=boolean  RndMeth=Simplest
  Constant : Constant  Value=0
  Constant1 : Constant  Value=0
  Cos : Trigonometry  Operator=cos
  Display{,1..4} (5 alike) : Display
  Divide : Product  Inputs=*/
  Divide1 : Product  Inputs=*/
  Gain : Gain  Gain=-2
  Gain1 : Gain  Gain=b_cx
  Gain2 : Gain  Gain=2
  Gain3 : Gain  Gain=g
  Gain4 : Gain  Gain=K_cy
  Gain5 : Gain  Gain=b_cy
  Integrator : Integrator
  Integrator1 : Integrator  InitialCondition=xt_inicial
  Integrator2 : Integrator
  Integrator3 : Integrator  InitialCondition=yl_inicial
  No entiendo para que : Constant  Value=0.1
  Product : Product
  Product1 : Product
  Sin : Trigonometry
  Sum : Sum  Inputs=|+-
  Sum1 : Sum  Inputs=|+-
  Sum2 : Sum  Inputs=++|
  Sum3 : Sum  Inputs=-+|
  Sum4 : Sum  Inputs=|+-
  Sum5 : Sum  Inputs=+-
  Sum6 : Sum  Inputs=|++
  Switch : Switch  Criteria=u2 > Threshold
  Switch1 : Switch  Criteria=u2 > Threshold
  Switch2 : Switch  Criteria=u2 > Threshold
  y_l - h_c <= y_co Carga apoyada : RelationalOperator  OutDataTypeStr=boolean  RndMeth=Simplest
  x_l : Outport
  y_l : Outport  Port=2
  d(x_xl) : Outport  Port=3
  d(y_l) : Outport  Port=4
  S_TLK : Outport  Port=5
  wires:
  F_hw/1 -> Display4/1, Gain2/1, Gain/1
  Theta/1 -> Display3/1, Cos/1, Sin/1
  Gain/1 -> Product/1
  Sin/1 -> Product/2
  Product/1 -> Sum/1
  Constant/1 -> Switch/1
  Gain1/1 -> Switch/3
  Switch/1 -> Sum/2
  Sum/1 -> Divide/1
  m_l/1 -> Divide/2, Display1/1, Divide1/2, Gain3/1
  Divide/1 -> Integrator/1  "dd(x_xl)"
  Integrator/1 -> Integrator1/1, d(x_xl)/1, Gain1/1  "d(x_xl)"
  Integrator1/1 -> x_l/1  "x_l"
  Cos/1 -> Product1/1
  Gain2/1 -> Product1/2
  Gain3/1 -> Sum1/2
  Product1/1 -> Sum1/1
  Constant1/1 -> Switch2/1, Switch1/1
  1/1 -> Switch2/2, Switch1/2, Switch/2
  Gain5/1 -> Switch2/3
  Gain4/1 -> Switch1/3
  Sum3/1 -> Display2/1, Divide1/1
  Switch2/1 -> Sum3/1
  Sum2/1 -> Sum3/2
  Sum1/1 -> Sum2/2
  Switch1/1 -> Sum2/1
  Integrator2/1 -> Gain5/1, d(y_l)/1, Integrator3/1  "d(y_l)"
  Divide1/1 -> Display/1, Integrator2/1  "dd(y_l)"
  Integrator3/1 -> Sum4/1, y_l/1  "y_l"
  h_c/1 -> Sum4/2
  Sum4/1 -> y_l - h_c <= y_co Carga apoyada/2, 1/1, Sum5/2
  Sum5/1 -> Gain4/1
  Y_co/1 -> 1/2, Sum5/1, Sum6/2
  No entiendo para que/1 -> Sum6/1
  Sum6/1 -> y_l - h_c <= y_co Carga apoyada/1
  y_l - h_c <= y_co Carga apoyada/1 -> S_TLK/1

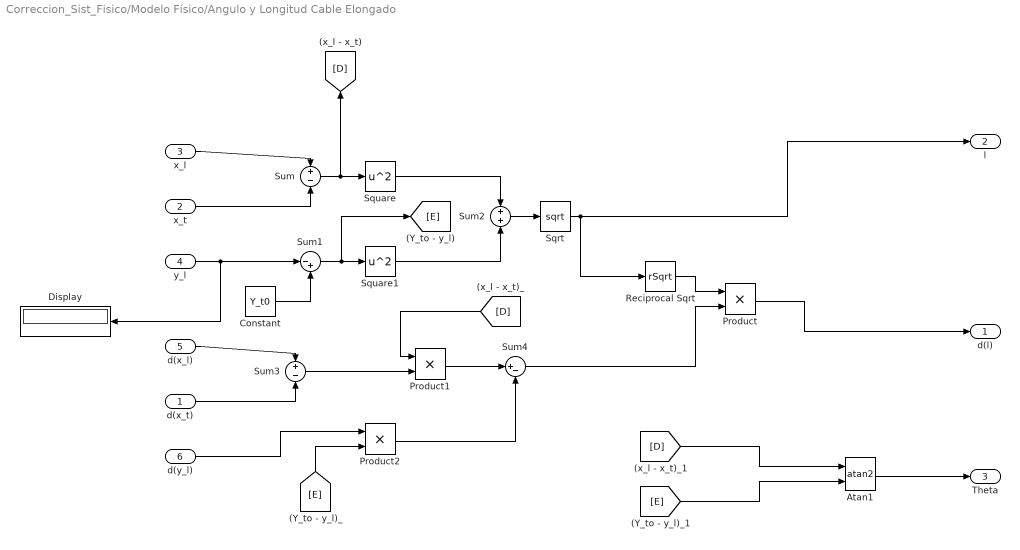
== system Correccion_Sist_Fisico/Modelo Físico/Angulo y Longitud Cable Elongado ==
  d(x_t) : Inport
  x_t : Inport  Port=2
  x_l : Inport  Port=3
  y_l : Inport  Port=4
  d(x_l) : Inport  Port=5
  d(y_l) : Inport  Port=6
  Atan1 : Trigonometry  Operator=atan2
  Constant : Constant  Value=Y_t0
  Display : Display
  Product : Product
  Product1 : Product
  Product2 : Product
  Reciprocal Sqrt : Sqrt  Operator=rSqrt  SaturateOnIntegerOverflow=on
  Sqrt : Sqrt  SaturateOnIntegerOverflow=on
  Square : Math  Operator=square  SaturateOnIntegerOverflow=on
  Square1 : Math  Operator=square  SaturateOnIntegerOverflow=on
  Sum : Sum  Inputs=+-
  Sum1 : Sum  Inputs=|-+
  Sum2 : Sum
  Sum3 : Sum  Inputs=+-
  Sum4 : Sum  Inputs=|+-
  d(l) : Outport
  l : Outport  Port=2
  Theta : Outport  Port=3
  wires:
  x_l/1 -> Sum/1
  x_t/1 -> Sum/2
  Sum/1 -> Square/1, [D]
  y_l/1 -> Display/1, Sum1/1
  Constant/1 -> Sum1/2
  Sum1/1 -> [E], Square1/1
  Square/1 -> Sum2/1
  Square1/1 -> Sum2/2
  Sum2/1 -> Sqrt/1
  Reciprocal Sqrt/1 -> Product/1
  Sqrt/1 -> Reciprocal Sqrt/1, l/1
  d(x_l)/1 -> Sum3/1
  d(x_t)/1 -> Sum3/2
  Sum3/1 -> Product1/2
  [D] -> Product1/1
  Product1/1 -> Sum4/1
  d(y_l)/1 -> Product2/1
  [E] -> Product2/2
  Product2/1 -> Sum4/2
  Sum4/1 -> Product/2
  Product/1 -> d(l)/1
  [E] -> Atan1/2
  Atan1/1 -> Theta/1
  [D] -> Atan1/1

== system Correccion_Sist_Fisico/Modelo Físico/Fines de carrera Carro ==
  x_t : Inport
  Aviso_Inferior : RelationalOperator  Operator=<=  OutDataTypeStr=boolean  RndMeth=Simplest
  Aviso_Superior : RelationalOperator  OutDataTypeStr=boolean  RndMeth=Simplest
  Constant : Constant  Value=50
  Constant1 : Constant  Value=-30
  Constant2 : Constant  Value=51
  Constant3 : Constant  Value=-31
  Limite_Inferior : RelationalOperator  Operator=<=  OutDataTypeStr=boolean  RndMeth=Simplest
  Limite_Superior : RelationalOperator  OutDataTypeStr=boolean  RndMeth=Simplest
  Lim_Sup : Outport
  Av_Sup : Outport  Port=2
  Lim_Inf : Outport  Port=3
  Av_Inf : Outport  Port=4
  wires:
  Constant/1 -> Limite_Superior/2
  Constant1/1 -> Limite_Inferior/2
  Constant2/1 -> Aviso_Superior/2
  Constant3/1 -> Aviso_Inferior/2
  x_t/1 -> Limite_Superior/1, Aviso_Superior/1, Limite_Inferior/1, Aviso_Inferior/1
  Aviso_Superior/1 -> Av_Sup/1
  Limite_Inferior/1 -> Lim_Inf/1
  Aviso_Inferior/1 -> Av_Inf/1
  Limite_Superior/1 -> Lim_Sup/1

== system Correccion_Sist_Fisico/Modelo Físico/Fines de carrera Izaje ==
  l : Inport
  Aviso_Inferior : RelationalOperator  Operator=<=  OutDataTypeStr=boolean  RndMeth=Simplest
  Aviso_Superior : RelationalOperator  OutDataTypeStr=boolean  RndMeth=Simplest
  Constant : Constant  Value=40
  Constant1 : Constant  Value=-20
  Constant2 : Constant  Value=41
  Constant3 : Constant  Value=-21
  Constant4 : Constant  Value=Y_t0
  Limite_Inferior : RelationalOperator  Operator=<=  OutDataTypeStr=boolean  RndMeth=Simplest
  Limite_Superior : RelationalOperator  OutDataTypeStr=boolean  RndMeth=Simplest
  x_h = Y_t0 - l_h : Sum  Inputs=|-+
  Lim_Sup : Outport
  Av_Sup : Outport  Port=2
  Lim_Inf : Outport  Port=3
  Av_Inf : Outport  Port=4
  wires:
  Limite_Inferior/1 -> Lim_Inf/1
  Constant/1 -> Limite_Superior/2
  Constant1/1 -> Limite_Inferior/2
  x_h = Y_t0 - l_h/1 -> Limite_Superior/1, Aviso_Superior/1, Limite_Inferior/1, Aviso_Inferior/1
  Limite_Superior/1 -> Lim_Sup/1
  Constant3/1 -> Aviso_Inferior/2
  Aviso_Inferior/1 -> Av_Inf/1
  Aviso_Superior/1 -> Av_Sup/1
  Constant2/1 -> Aviso_Superior/2
  l/1 -> x_h = Y_t0 - l_h/1
  Constant4/1 -> x_h = Y_t0 - l_h/2

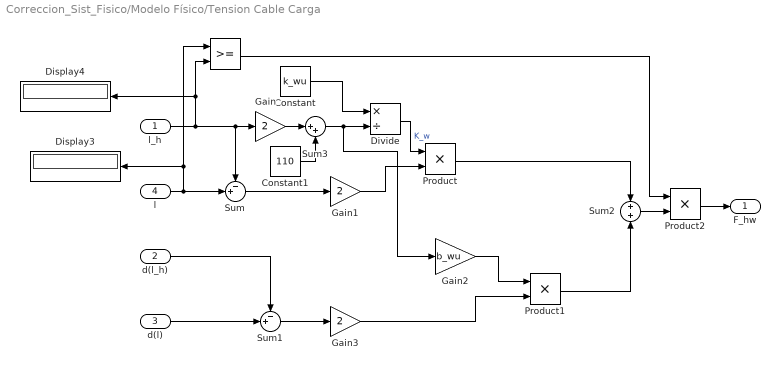
== system Correccion_Sist_Fisico/Modelo Físico/Tension Cable Carga ==
  l_h : Inport
  d(l_h) : Inport  Port=2
  d(l) : Inport  Port=3
  l : Inport  Port=4
  " " : RelationalOperator  OutDataTypeStr=boolean  RndMeth=Simplest
  Constant : Constant  Value=k_wu
  Constant1 : Constant  Value=110
  Display3 : Display
  Display4 : Display
  Divide : Product  Inputs=*/
  Gain : Gain  Gain=2
  Gain1 : Gain  Gain=2
  Gain2 : Gain  Gain=b_wu
  Gain3 : Gain  Gain=2
  Product : Product
  Product1 : Product
  Product2 : Product
  Sum : Sum  Inputs=-+|
  Sum1 : Sum  Inputs=-+|
  Sum2 : Sum
  Sum3 : Sum  Inputs=|++
  F_hw : Outport
  wires:
  l_h/1 -> Gain/1, Sum/1, Display4/1, " "/2
  Sum/1 -> Gain1/1
  Gain1/1 -> Product/2
  d(l)/1 -> Sum1/2
  d(l_h)/1 -> Sum1/1
  Sum1/1 -> Gain3/1
  Gain2/1 -> Product1/1
  Gain3/1 -> Product1/2
  Product/1 -> Sum2/1
  Product1/1 -> Sum2/2
  Constant/1 -> Divide/1
  Gain/1 -> Sum3/1
  Sum3/1 -> Gain2/1, Divide/2
  Constant1/1 -> Sum3/2
  Divide/1 -> Product/1  "K_w"
  l/1 -> Display3/1, " "/1, Sum/2
  Sum2/1 -> Product2/2
  Product2/1 -> F_hw/1
  " "/1 -> Product2/1

== system Correccion_Sist_Fisico/Modelo Físico/Tension Cable Carro ==
  x_td : Inport
  dx_td : Inport  Port=2
  x_t : Inport  Port=3
  dx_t : Inport  Port=4
  Gain : Gain  Gain=K_tw
  Gain1 : Gain  Gain=b_tw
  Sum : Sum  Inputs=+-
  Sum1 : Sum  Inputs=+-
  Sum2 : Sum
  F_tw : Outport
  wires:
  x_td/1 -> Sum/1
  x_t/1 -> Sum/2
  Sum/1 -> Gain/1
  Sum1/1 -> Gain1/1
  dx_td/1 -> Sum1/1
  dx_t/1 -> Sum1/2
  Gain/1 -> Sum2/1
  Gain1/1 -> Sum2/2
  Sum2/1 -> F_tw/1

== system Correccion_Sist_Fisico/Modelo Físico/Traslacion Carro ==
  F_tw : Inport
  F_hw : Inport  Port=2
  Theta : Inport  Port=3
  Gain : Gain  Gain=2
  Gain1 : Gain  Gain=1/M_t
  Gain2 : Gain  Gain=b_t
  Integrator : Integrator
  Integrator1 : Integrator  InitialCondition=xt_inicial
  Product : Product
  Sin : Trigonometry
  Sum : Sum  Inputs=++-
  X_t : Outport
  d(X_t) : Outport  Port=2
  wires:
  Theta/1 -> Sin/1
  Sin/1 -> Product/2
  F_hw/1 -> Product/1
  Product/1 -> Gain/1
  Gain/1 -> Sum/2
  F_tw/1 -> Sum/1
  Sum/1 -> Gain1/1
  Gain1/1 -> Integrator/1  "dd(X_t)"
  Integrator/1 -> d(X_t)/1, Gain2/1, Integrator1/1  "d(X_t)"
  Gain2/1 -> Sum/3
  Integrator1/1 -> X_t/1

== system Correccion_Sist_Fisico/Modelo Físico/TwistLock ==
  TLK : Inport
  M_Cx : Inport  Port=2
  Chart : Stateflow chart  TreatAsAtomicUnit=on
  Chart1 : Stateflow chart  TreatAsAtomicUnit=on
  Display{,1..3} (4 alike) : Display
  m_l : Outport
  h_c : Outport  Port=2
  wires:
  Chart/1(m_l) -> Display/1, m_l/1
  Chart/2(h_c) -> h_c/1, Display1/1
  M_Cx/1 -> Chart1/2(M_Cx), Chart/2(M_Cx)
  Chart1/1(m_l) -> Display2/1
  Chart1/2(h_c) -> Display3/1
  TLK/1 -> Chart1/1(TLK), Chart/1(TLK)

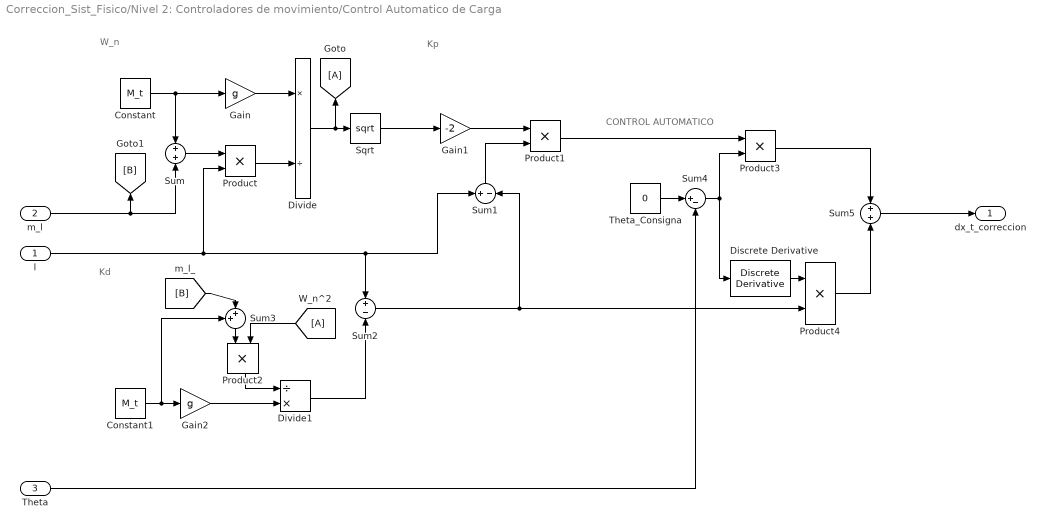
== system Correccion_Sist_Fisico/Nivel 2: Controladores de movimiento/Control Automatico de Carga ==
  note: CONTROL AUTOMATICO
  note: Kd
  note: Kp
  note: W_n
  l : Inport
  m_l : Inport  Port=2
  Theta : Inport  Port=3
  Constant : Constant  Value=M_t
  Constant1 : Constant  Value=M_t
  Discrete Derivative : simulink/Discrete/Discrete Derivative  gainval=1.0  ICPrevScaledInput=0.0  OutMin=[]  OutMax=[]  OutDataType=fixdt(1, 16)  OutScaling=2^-10  DoSatur=off
  Divide : Product  Inputs=*/
  Divide1 : Product  Inputs=/*
  Gain : Gain  Gain=g
  Gain1 : Gain  Gain=-2
  Gain2 : Gain  Gain=g
  Product{,1..4} (5 alike) : Product
  Sqrt : Sqrt  SaturateOnIntegerOverflow=on
  Sum : Sum
  Sum1 : Sum  Inputs=+-
  Sum2 : Sum  Inputs=+-
  Sum3 : Sum  Inputs=++|
  Sum4 : Sum  Inputs=|+-
  Sum5 : Sum
  Theta_Consigna : Constant  Value=0
  dx_t_correccion : Outport
  wires:
  Constant/1 -> Sum/1, Gain/1
  Gain/1 -> Divide/1
  m_l/1 -> [B], Sum/2
  Sum/1 -> Product/1
  l/1 -> Sum1/1, Sum2/1, Product/2
  Product/1 -> Divide/2
  Divide/1 -> [A], Sqrt/1
  Sqrt/1 -> Gain1/1
  Gain1/1 -> Product1/1
  Sum1/1 -> Product1/2
  Constant1/1 -> Sum3/1, Gain2/1
  Gain2/1 -> Divide1/2
  Sum3/1 -> Product2/1
  Product2/1 -> Divide1/1
  [A] -> Product2/2
  [B] -> Sum3/2
  Divide1/1 -> Sum2/2
  Sum2/1 -> Product4/2, Sum1/2
  Theta_Consigna/1 -> Sum4/1
  Theta/1 -> Sum4/2
  Product1/1 -> Product3/1
  Sum4/1 -> Discrete Derivative/1, Product3/2
  Product3/1 -> Sum5/1
  Discrete Derivative/1 -> Product4/1
  Product4/1 -> Sum5/2
  Sum5/1 -> dx_t_correccion/1

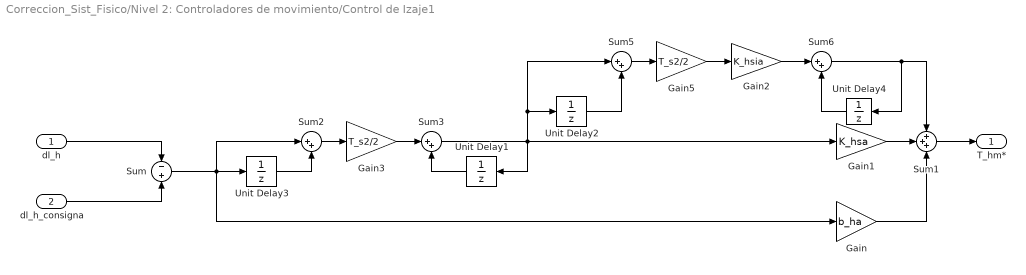
== system Correccion_Sist_Fisico/Nivel 2: Controladores de movimiento/Control de Izaje1 ==
  dl_h : Inport
  dl_h_consigna : Inport  Port=2
  Gain : Gain  Gain=b_ha
  Gain1 : Gain  Gain=K_hsa
  Gain2 : Gain  Gain=K_hsia
  Gain3 : Gain  Gain=T_s2/2
  Gain5 : Gain  Gain=T_s2/2
  Sum : Sum  Inputs=-+
  Sum1 : Sum  Inputs=+++
  Sum{2..3,5..6} (4 alike) : Sum  Inputs=|++
  Unit Delay{1..4} (4 alike) : UnitDelay  SampleTime=-1  HasFrameUpgradeWarning=on
  T_hm* : Outport
  wires:
  Unit Delay4/1 -> Sum6/2
  Sum3/1 -> Unit Delay1/1, Gain1/1, Unit Delay2/1, Sum5/1
  Sum5/1 -> Gain5/1
  Gain5/1 -> Gain2/1
  Unit Delay2/1 -> Sum5/2
  Unit Delay1/1 -> Sum3/2
  Gain3/1 -> Sum3/1
  Sum2/1 -> Gain3/1
  Unit Delay3/1 -> Sum2/2
  Gain1/1 -> Sum1/2
  Sum1/1 -> T_hm*/1
  dl_h_consigna/1 -> Sum/2
  Sum/1 -> Unit Delay3/1, Gain/1, Sum2/1
  dl_h/1 -> Sum/1
  Sum6/1 -> Sum1/1, Unit Delay4/1
  Gain/1 -> Sum1/3
  Gain2/1 -> Sum6/1

== system Correccion_Sist_Fisico/Nivel 2: Controladores de movimiento/Control de Traslacion ==
  dx_td : Inport
  dx_td_consigna : Inport  Port=2
  Gain : Gain  Gain=b_ta
  Gain1 : Gain  Gain=K_tsa
  Gain2 : Gain  Gain=K_tsia
  Gain3 : Gain  Gain=T_s2/2
  Gain5 : Gain  Gain=T_s2/2
  Sum : Sum  Inputs=-+
  Sum1 : Sum  Inputs=+++
  Sum{2..3,5..6} (4 alike) : Sum  Inputs=|++
  Unit Delay{1..3,7} (4 alike) : UnitDelay  SampleTime=-1  HasFrameUpgradeWarning=on
  T_tm* : Outport
  wires:
  Gain/1 -> Sum1/3
  dx_td/1 -> Sum/1
  Sum/1 -> Unit Delay7/1, Sum2/1, Gain/1
  dx_td_consigna/1 -> Sum/2
  Sum1/1 -> T_tm*/1
  Gain1/1 -> Sum1/2
  Unit Delay7/1 -> Sum2/2
  Sum2/1 -> Gain3/1
  Gain3/1 -> Sum3/1
  Unit Delay1/1 -> Sum3/2
  Unit Delay2/1 -> Sum5/2
  Sum5/1 -> Gain5/1
  Sum3/1 -> Unit Delay1/1, Unit Delay2/1, Sum5/1, Gain1/1
  Unit Delay3/1 -> Sum6/2
  Gain5/1 -> Gain2/1
  Sum6/1 -> Sum1/1, Unit Delay3/1
  Gain2/1 -> Sum6/1

== system Correccion_Sist_Fisico/Nivel 2: Controladores de movimiento/Control de Traslacion1 ==
  dx_td : Inport
  dx_td_consigna : Inport  Port=2
  Discrete-Time Integrator : DiscreteIntegrator  SampleTime=T_s2  ICPrevOutput=DiscIntNeverNeededParam  ICPrevScaledInput=DiscIntNeverNeededParam
  Discrete-Time Integrator1 : DiscreteIntegrator  SampleTime=T_s2  ICPrevOutput=DiscIntNeverNeededParam  ICPrevScaledInput=DiscIntNeverNeededParam
  Gain : Gain  Gain=b_ta
  Gain1 : Gain  Gain=K_tsa
  Gain2 : Gain  Gain=K_tsia
  Sum : Sum  Inputs=-+
  Sum1 : Sum  Inputs=+++
  T_tm* : Outport
  wires:
  Gain/1 -> Sum1/3
  dx_td/1 -> Sum/1
  Sum/1 -> Discrete-Time Integrator/1, Gain/1
  dx_td_consigna/1 -> Sum/2
  Sum1/1 -> T_tm*/1
  Gain1/1 -> Sum1/2
  Discrete-Time Integrator1/1 -> Gain2/1
  Gain2/1 -> Sum1/1
  Discrete-Time Integrator/1 -> Discrete-Time Integrator1/1, Gain1/1

== system Correccion_Sist_Fisico/Nivel 2: Controladores de movimiento/Estimación de l ==
  F_hw : Inport
  l_h : Inport  Port=2
  Constant : Constant  Value=110
  Constant1 : Constant  Value=k_wu
  Divide : Product  Inputs=*/
  Divide1 : Product  Inputs=*/
  Gain1 : Gain  Gain=2
  Gain2 : Gain  Gain=1/2
  Memory2 : Memory
  Sum1 : Sum  Inputs=|++
  Sum3 : Sum  Inputs=|++
  l^ : Outport
  wires:
  Constant/1 -> Sum3/2
  Divide/1 -> Divide1/2  "K_w"
  l_h/1 -> Sum1/2, Gain1/1  "l_h"
  Sum3/1 -> Divide/2
  Gain1/1 -> Sum3/1
  Constant1/1 -> Divide/1
  F_hw/1 -> Divide1/1
  Divide1/1 -> Gain2/1  "K_w"
  Gain2/1 -> Sum1/1  "1/2 F_hw/Kw"
  Sum1/1 -> Memory2/1
  Memory2/1 -> l^/1

== system Correccion_Sist_Fisico/JOYSTICK/Movimiento Carro e Izaje/Sensibilidad1 ==
  Analogo_IZQ_Vertical : Inport
  Analogo_DER_Horizontal : Inport  Port=2
  Compare To Constant : simulink/Logic and Bit Operations/Compare To Constant  relop=>=  const=0.15  OutDataTypeStr=boolean
  Compare To Constant1 : simulink/Logic and Bit Operations/Compare To Constant  relop=<=  const=-0.15  OutDataTypeStr=boolean
  Compare To Constant2 : simulink/Logic and Bit Operations/Compare To Constant  relop=>=  const=0.15  OutDataTypeStr=boolean
  Compare To Constant3 : simulink/Logic and Bit Operations/Compare To Constant  relop=<=  const=-0.15  OutDataTypeStr=boolean
  OR : Logic  Operator=OR  IconShape=distinctive  AllPortsSameDT=off  OutDataTypeStr=boolean
  OR1 : Logic  Operator=OR  IconShape=distinctive  AllPortsSameDT=off  OutDataTypeStr=boolean
  Product : Product
  Product1 : Product
  V_max_CARRO : Gain  Gain=4
  V_max_IZAJE : Gain  Gain=3
  dl_h_ref_manual : Outport
  dx_t_ref_man : Outport  Port=2
  wires:
  Analogo_IZQ_Vertical/1 -> V_max_IZAJE/1
  Analogo_DER_Horizontal/1 -> V_max_CARRO/1
  Compare To Constant1/1 -> OR/2
  Compare To Constant2/1 -> OR1/1
  Compare To Constant3/1 -> OR1/2
  OR1/1 -> Product1/1
  Compare To Constant/1 -> OR/1
  OR/1 -> Product/1
  Product/1 -> dl_h_ref_manual/1
  Product1/1 -> dx_t_ref_man/1
  V_max_CARRO/1 -> Product1/2, Compare To Constant2/1, Compare To Constant3/1
  V_max_IZAJE/1 -> Compare To Constant/1, Compare To Constant1/1, Product/2

== matlab function Correccion_Sist_Fisico/MATLAB Function ==
  data: masa input; velocidad_maxima output; estable input
function velocidad_maxima = calcular_velocidad_maxima_Izaje(masa, estable)
    % Puntos conocidos (masa, velocidad)
    if (estable)
        puntos_conocidos = [
            65000, 1.5;
            60000, 1.67;
            53000, 1.83;
            50000, 1.9;
            48000, 2;
            45000, 2.1;
            44000, 2.166;
            41000, 2.33;
            40000, 2.4;
            38000, 2.5;
            35000, 2.7;
            34000, 2.88;
            32000, 3;
            30000, 3;
            25000, 3;
            20000, 3;
            15000, 3
        ];

        % Realizar interpolación lineal
        velocidad_maxima = interp1(puntos_conocidos(:, 1), puntos_conocidos(:, 2), masa, 'linear');

        % Asegurarse de que la velocidad no sea NaN si la masa está fuera del rango
        if isnan(velocidad_maxima)
            velocidad_maxima = 0;
        end
    else
        velocidad_maxima = 2;
    end
    
end

== stateflow chart Correccion_Sist_Fisico/JOYSTICK/Mantener Seleccion ==
  state Espera
  state Invertir
    entry:
    X_=(~X_);
  (default) -> Espera
  Espera -> Invertir : [X~=0]
  Invertir -> Espera : [X==0]
  data: X input; X_ output boolean =false

== stateflow chart Correccion_Sist_Fisico/JOYSTICK/Mantener Seleccion1 ==
  state Espera
  state Invertir
    entry:
    Select_=(~Select_);
  (default) -> Espera
  Espera -> Invertir : [Select~=0]
  Invertir -> Espera : [Select==0]
  data: Select input; Select_ output boolean =false

== stateflow chart Correccion_Sist_Fisico/JOYSTICK/Mantener Seleccion2 ==
  state Espera
  state Invertir
    entry:
    a_=(~a_);
  (default) -> Espera
  Espera -> Invertir : [a~=0]
  Invertir -> Espera : [a==0]
  data: a input; a_ output boolean =false

== stateflow chart Correccion_Sist_Fisico/JOYSTICK/Mantener Seleccion3 ==
  state Espera
  state Invertir
    entry:
    L1_=(~L1_);
  (default) -> Espera
  Espera -> Invertir : [L1~=0]
  Invertir -> Espera : [L1==0]
  data: L1 input; L1_ output boolean =false

== stateflow chart Correccion_Sist_Fisico/JOYSTICK/Mantener Seleccion4 ==
  state Espera
  state Invertir
    entry:
    R1_=(~R1_);
  (default) -> Espera
  Espera -> Invertir : [R1~=0]
  Invertir -> Espera : [R1==0]
  data: R1 input; R1_ output boolean =false

== stateflow chart Correccion_Sist_Fisico/Modelo Físico/TwistLock/Chart1 ==
  state OFF
    m_l = M_s;
    h_c = 0;
  state ON
    m_l = M_s + M_Cx;
    h_c = H_c;
  (default) -> OFF
  OFF -> ON : [TLK == 1]
  ON -> OFF : [TLK == 0]
  data: TLK input; M_Cx input; m_l output; h_c output; H_c parameter; M_s parameter

== stateflow chart Correccion_Sist_Fisico/Modelo Físico/TwistLock/Chart ==
  (default) -> (junction 14)
  (junction 14) -> (junction 16) [order 1] : [~TLK]
  (junction 14) -> (junction 18) [order 2] : {m_l = M_s + M_Cx; h_c  = H_c}
  (junction 16) -> (junction 20) : {m_l = M_s; h_c =0}
  (junction 20) -> (junction 18)
  (junction 18) -> (junction 23)
  data: TLK input; M_Cx input; m_l output; h_c output; H_c parameter; M_s parameter

== stateflow chart Correccion_Sist_Fisico/Chart1 ==
  state PosicionesContenedores
    entry:
    % Esta es la forma que econtré para que llame
    % la función solo una vez
    posiciones_contenedor = generar_obstaculos();
  (default) -> PosicionesContenedores
  data: contenedor_pos function_output; posiciones_contenedor output
  function contenedor_pos  = generar_obstaculos:
    | function contenedor_pos  = generar_obstaculos
    |     % Inicializar la figura
    |     figure;
    |     hold on;
    |     xlabel('x');
    |     ylabel('y');
    |     grid on;
    |     axis([-35, 55, -20, 50]);
    | 
    |     % Izaje
    |     x_izaje = -35:55;
    |     yt0 = ones(size(x_izaje)) * 45;
    |     plot(x_izaje, yt0, '*b');
    | 
    |     % Muelle
    |     % Línea horizontal
    |     x_muelle_h = -35:0;
    |     y_muelle_h = zeros(size(x_muelle_h));
    |     plot(x_muelle_h, y_muelle_h, 'k', 'LineWidth', 2);
    | 
    |     % Línea vertical
    |     y_muelle_v = -20:0;
    |     x_muelle_v = zeros(size(y_muelle_v));
    |     plot(x_muelle_v, y_muelle_v, 'k', 'LineWidth', 2);
    | 
    |     % Barco
    |     % Horizontal abajo
    |     x_barco_h_a = 2.5:50;
    |     y_barco_h_a = ones(size(x_barco_h_a)) * -20;
    |     plot(x_barco_h_a, y_barco_h_a, 'y', 'LineWidth', 4);
    | 
    |     % Horizontal izquierda
    |     x_barco_h_i = 0:2.5;
    |     y_barco_h_i = zeros(size(x_barco_h_i));
    |     plot(x_barco_h_i, y_barco_h_i, 'y', 'LineWidth', 4);
    | 
    |     % Vertical izquierda
    |     y_barco_v = -20:0;
    |     x_barco_v_i = ones(size(y_muelle_v)) * 2.5;
    |     plot(x_barco_v_i, y_barco_v, 'y', 'LineWidth', 4);
    | 
    |     % Vertical derecha
    |     x_barco_v_d = ones(size(y_muelle_v)) * 50;
    |     plot(x_barco_v_d, y_barco_v, 'y', 'LineWidth', 4);
    | 
    |     % Contenedores dentro del barco
    |     num_columnas = 16;
    |     num_contenedores_min = 10;
    |     num_contenedores_max = 18;
    | 
    |     contenedor_pos = zeros(num_contenedores_max, num_columnas);
    | 
    |     for columna = 1:num_columnas
    |         % Dibujo de todos los contenedores en la fila actual
    |         num_contenedores_fila = randi([num_contenedores_min, num_contenedores_max]);
    |         posiciones_fila = zeros(num_contenedores_fila, 2);
    | 
    |         for i = 1:num_contenedores_fila
    |             contenedor_pos(i,columna) = 1;
    |             
    |             % ------------ Para graficar -------------
    |             pos_x = 2.5 + (columna - 1) * 3;
    |             pos_y = -20 + (i - 1) * 2.5;
    |             % Almacena la posición del contenedor
    |             posiciones_fila(i, :) = [pos_x, pos_y];
    |             
    |             % Dibuja el contenedor
    |             rectangle('Position', [pos_x, pos_y, 2.5, 2.5], 'EdgeColor', 'r', 'LineWidth', 2);
    |             % Etiqueta 'x' en el centro del contenedor
    |             x_center = pos_x + 1.25;
    |             y_center = pos_y + 1.25;
    |             text(x_center, y_center, 'x', 'Color', 'r', 'FontSize', 12, 'HorizontalAlignment', 'center', 'VerticalAlignment', 'middle');
    |         end
    |         
    |     end
    | end
